simulink model "ClosedLoop_Cq"  (R2023b)
settings: Solver=VariableStepAuto  StartTime=0.0  StopTime=10.0  RelTol=1e-3
libraries: cstblocks x3
settings Model: Creator=bolee  LastModifiedBy=bolee

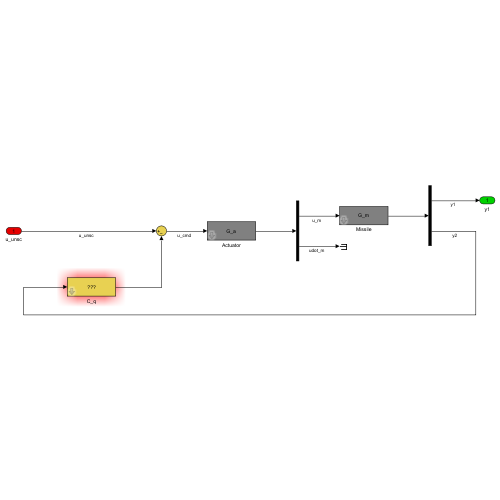
[thumbnail: Simulink's stored preview of the top-level diagram]
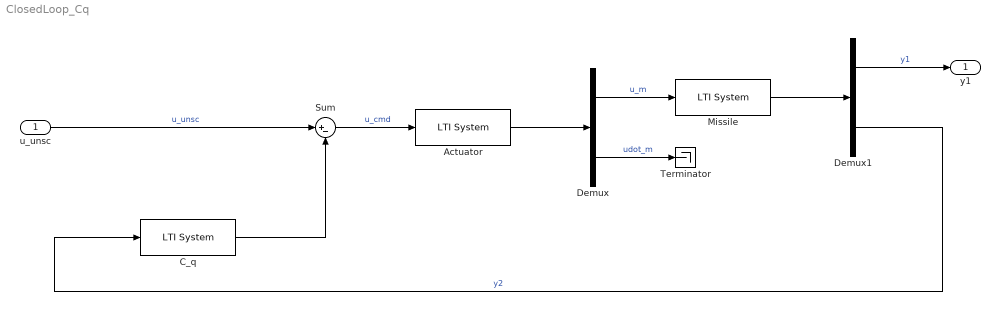
== system ClosedLoop_Cq ==
  u_unsc : Inport
  Actuator : cstblocks/LTI System  sys=G_a  IC=[]  PadeOrder=0
  C_q : cstblocks/LTI System  sys=C_q  IC=[]  PadeOrder=0
  Demux : Demux  Outputs=2
  Demux1 : Demux  Outputs=2
  Missile : cstblocks/LTI System  sys=G_m  IC=[]  PadeOrder=0
  Sum : Sum  Inputs=|+-
  Terminator : Terminator
  y1 : Outport
  wires:
  Actuator/1 -> Demux/1
  Sum/1 -> Actuator/1  "u_cmd"
  Demux/1 -> Missile/1  "u_m"
  Demux/2 -> Terminator/1  "udot_m"
  Missile/1 -> Demux1/1
  Demux1/2 -> C_q/1  "y2"
  Demux1/1 -> y1/1  "y1"
  C_q/1 -> Sum/2
  u_unsc/1 -> Sum/1  "u_unsc"
